simulink model "NivelTanque"  (R2024b)
settings: Solver=VariableStepAuto  StartTime=0.0  StopTime=10.0  RelTol=1e-3
undefined symbols (not defined in the file): DiscIntNeverNeededParam
libraries: simulink x1
settings Model: Creator=Msi  LastModifiedBy=Msi
settings OptimizationCC: OptimizeBlockIOStorage=off
settings RTWCC: BuildConfiguration=Debug
settings CodeAppCC: ForceParamTrailComments=on  MATLABSourceComments=on

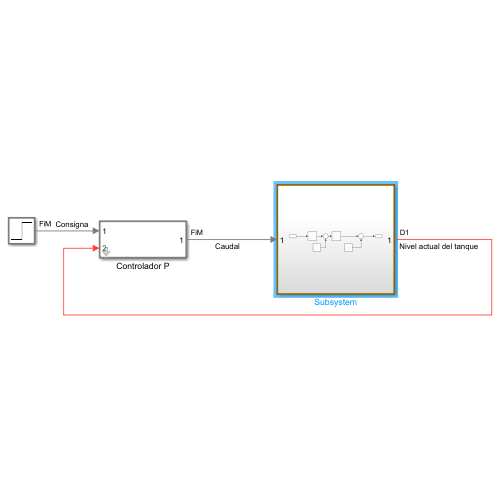
[thumbnail: Simulink's stored preview of the top-level diagram]
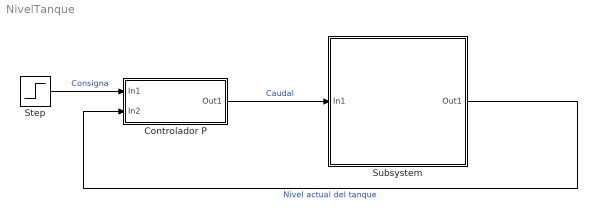
== system NivelTanque ==
  Controlador P : Subsystem  mask{Kp=5}
      mask prompts: Kp "Variable proporcional"
  Step : Step  SampleTime=0
  Subsystem : Subsystem
  wires:
  Controlador P/1(Out1) -> Subsystem/1(In1)  "Caudal"
  Step/1 -> Controlador P/1(In1)  "Consigna"
  Subsystem/1(Out1) -> Controlador P/2(In2)  "Nivel actual del tanque"

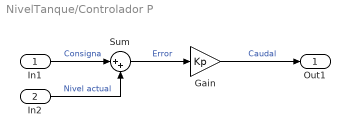
== system NivelTanque/Controlador P ==
  In1 : Inport
  In2 : Inport  Port=2
  Gain : Gain  Gain=Kp
  Sum : Sum  Inputs=|++
  Out1 : Outport
  wires:
  In1/1 -> Sum/1  "Consigna"
  Gain/1 -> Out1/1  "Caudal"
  In2/1 -> Sum/2  "Nivel actual"
  Sum/1 -> Gain/1  "Error"

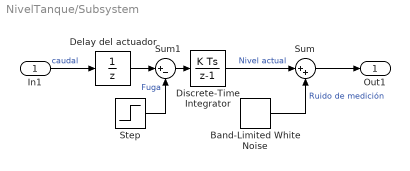
== system NivelTanque/Subsystem ==
  In1 : Inport
  Band-Limited White Noise : simulink/Sources/Band-Limited White Noise  Cov=[0.1]  Ts=1/1000  seed=[23341]
  Delay del actuador : UnitDelay  SampleTime=1/1000  HasFrameUpgradeWarning=on
  Discrete-Time Integrator : DiscreteIntegrator  SampleTime=1/1000  ICPrevOutput=DiscIntNeverNeededParam  ICPrevScaledInput=DiscIntNeverNeededParam
  Step : Step  SampleTime=0
  Sum : Sum  Inputs=|++
  Sum1 : Sum  Inputs=|+-
  Out1 : Outport
  wires:
  In1/1 -> Delay del actuador/1  "caudal"
  Discrete-Time Integrator/1 -> Sum/1  "Nivel actual"
  Sum/1 -> Out1/1
  Band-Limited White Noise/1 -> Sum/2  "Ruido de medición"
  Delay del actuador/1 -> Sum1/1
  Sum1/1 -> Discrete-Time Integrator/1
  Step/1 -> Sum1/2  "Fuga"
